simulink model "idF14Model"  (R2016a)
settings: Solver=ode45  SolverMode=SingleTasking  StartTime=0.0  StopTime=30  RelTol=1e-4  AbsTol=1e-6
PreLoadFcn:
  | g = 32.2;
  | Uo = 689.4000;
  | Vto = 690.4000;
  | % Stability derivatives
  | Mw = -0.00592;
  | Mq = -0.6571;
  | Md = -6.8847;
  | Zd = -63.9979;
  | Zw = -0.6385;
  | % Gains
  | cmdgain = 3.490954472728077e-02;
  | Ka = 0.6770;
  | Kq = 0.8156;
  | Kf = -1.7460;
  | Ki = -3.8640;
  | % Other constants
  | a = 2.5348;
  | Gamma = 0.0100;
  | b = 64.1300;
  | Beta = 426.4352;
  | Sa = 0.005236;
  | Swg = 3;
  | Ta = 0.0500;
  | Tal = 0.3959;
  | Ts = 0.0444;
  | W1 = 2.9710;
  | W2 = 4.1440;
  | Wa = 10;
libraries: simulink x1
settings Model: ExtModeTrigMode=oneshot  ExtModeArmWhenConnect=off  ExtModeAutoUpdateStatusClock=off  Creator=The MathWorks, Inc.  LastModifiedBy=The MathWorks, Inc.
settings DataIOCC: ExternalInput=[]  InitialState=[]  SaveFormat=Array  SaveOutput=off  SaveTime=off
settings OptimizationCC: BlockReduction=off  BooleanDataType=off  ExpressionDepthLimit=2147483647  InitFltsAndDblsToZero=on
settings DebuggingCC: SaveWithParameterizedLinksMsg=none  UnderspecifiedInitializationDetection=Classic  MergeDetectMultiDrivingBlocksExec=none  SignalResolutionControl=TryResolveAllWithWarning  MultiTaskDSMMsg=warning  MultiTaskCondExecSysMsg=none  IntegerOverflowMsg=none  FcnCallInpInsideContextMsg=UseLocalSettings  StateNameClashWarn=warning  IntegerSaturationMsg=none
settings HardwareCC: ProdBitPerPointer=32  ProdLargestAtomicFloat=None  ProdIntDivRoundTo=Undefined  ProdEndianess=Unspecified  ProdWordSize=32  ProdHWDeviceType=32-bit Generic
settings ModelReferenceCC: PropagateSignalLabelsOutOfModel=off
settings GRTTargetCC: TargetFcnLib=ansi_tfl_tmw.mat  CombineOutputUpdateFcns=off  GRTInterface=on
settings ConfigComp: CovModelRefEnable=Off

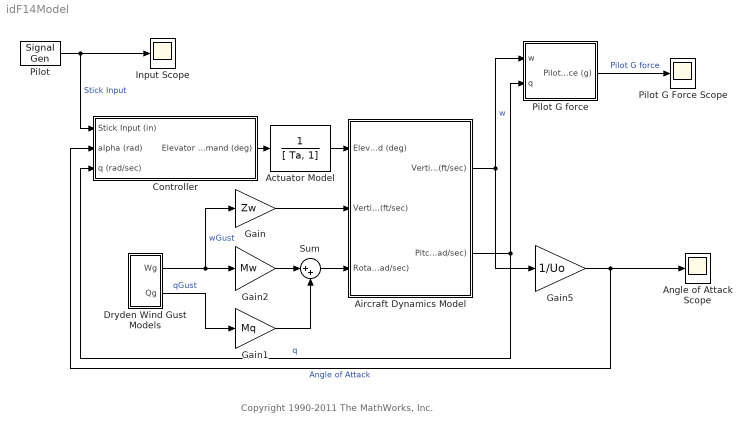
== system idF14Model ==
  note: Copyright 1990-2011 The MathWorks, Inc.
  Actuator Model : TransferFcn  Denominator=[ Ta, 1]
  Aircraft Dynamics Model : Subsystem
  Angle of Attack Scope : Scope
  Controller : Subsystem
  Dryden Wind Gust Models : Subsystem
  Gain : Gain  Gain=Zw  SaturateOnIntegerOverflow=on  OutDataTypeStr=Inherit: Same as input  ParamDataTypeStr=Inherit: Same as input
  Gain1 : Gain  Gain=Mq  SaturateOnIntegerOverflow=on  OutDataTypeStr=Inherit: Same as input  ParamDataTypeStr=Inherit: Same as input
  Gain2 : Gain  Gain=Mw  SaturateOnIntegerOverflow=on  OutDataTypeStr=Inherit: Same as input  ParamDataTypeStr=Inherit: Same as input
  Gain5 : Gain  Gain=1/Uo  SaturateOnIntegerOverflow=on  OutDataTypeStr=Inherit: Same as input  ParamDataTypeStr=Inherit: Same as input
  Input Scope : Scope
  Pilot : SignalGenerator  WaveForm=square  Frequency=0.500000  Units=rad/sec
  Pilot G Force Scope : Scope
  Pilot G force : Subsystem
  Sum : Sum  Inputs=|++  SaturateOnIntegerOverflow=on  InputSameDT=on  OutDataTypeStr=Inherit: Same as first input
  wires:
  Gain5/1 -> Angle of Attack Scope/1, Controller/2(alpha (rad))  "Angle of Attack"
  Aircraft Dynamics Model/1(Vertical Velocity w (ft/sec)) -> Gain5/1, Pilot G force/1(w)  "w"
  Pilot G force/1(Pilot g force (g)) -> Pilot G Force Scope/1  "Pilot G force"
  Gain2/1 -> Sum/1
  Gain/1 -> Aircraft Dynamics Model/2(Vertical Gust wGust (ft/sec))
  Dryden Wind Gust Models/2(Qg) -> Gain1/1  "qGust"
  Dryden Wind Gust Models/1(Wg) -> Gain2/1, Gain/1  "wGust"
  Sum/1 -> Aircraft Dynamics Model/3(Rotary Gust qGust (rad/sec))
  Gain1/1 -> Sum/2
  Aircraft Dynamics Model/2(Pitch Rate q (rad/sec)) -> Pilot G force/2(q), Controller/3(q (rad/sec))  "q"
  Actuator Model/1 -> Aircraft Dynamics Model/1(Elevator Deflection d (deg))
  Controller/1(Elevator Command (deg)) -> Actuator Model/1
  Pilot/1 -> Input Scope/1, Controller/1(Stick Input (in))  "Stick Input"

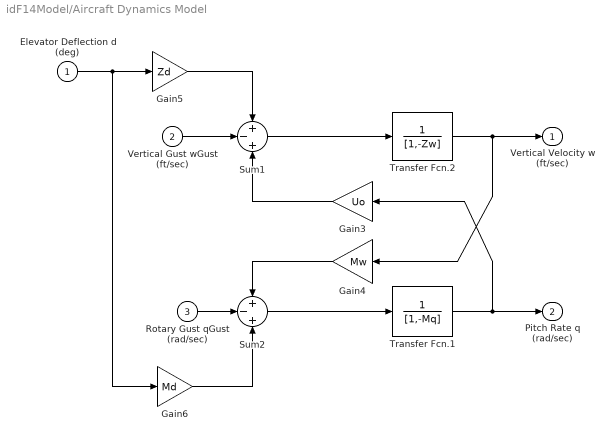
== system idF14Model/Aircraft Dynamics Model ==
  Elevator Deflection d (deg) : Inport
  Vertical Gust wGust (ft/sec) : Inport  Port=2
  Rotary Gust qGust (rad/sec) : Inport  Port=3
  Gain3 : Gain  Gain=Uo  SaturateOnIntegerOverflow=on  OutDataTypeStr=Inherit: Same as input  ParamDataTypeStr=Inherit: Same as input
  Gain4 : Gain  Gain=Mw  SaturateOnIntegerOverflow=on  OutDataTypeStr=Inherit: Same as input  ParamDataTypeStr=Inherit: Same as input
  Gain5 : Gain  Gain=Zd  SaturateOnIntegerOverflow=on  OutDataTypeStr=Inherit: Same as input  ParamDataTypeStr=Inherit: Same as input
  Gain6 : Gain  Gain=Md  SaturateOnIntegerOverflow=on  OutDataTypeStr=Inherit: Same as input  ParamDataTypeStr=Inherit: Same as input
  Sum1 : Sum  Inputs=+-+  SaturateOnIntegerOverflow=on  InputSameDT=on  OutDataTypeStr=Inherit: Same as first input
  Sum2 : Sum  Inputs=+-+  SaturateOnIntegerOverflow=on  InputSameDT=on  OutDataTypeStr=Inherit: Same as first input
  Transfer Fcn.1 : TransferFcn  Denominator=[1,-Mq]
  Transfer Fcn.2 : TransferFcn  Denominator=[1,-Zw]
  Vertical Velocity w (ft/sec) : Outport  InitialOutput=0
  Pitch Rate q (rad/sec) : Outport  Port=2  InitialOutput=0
  wires:
  Transfer Fcn.2/1 -> Vertical Velocity w (ft/sec)/1, Gain4/1
  Transfer Fcn.1/1 -> Pitch Rate q (rad/sec)/1, Gain3/1
  Gain6/1 -> Sum2/3
  Gain5/1 -> Sum1/1
  Gain3/1 -> Sum1/3
  Rotary Gust qGust (rad/sec)/1 -> Sum2/2
  Sum2/1 -> Transfer Fcn.1/1
  Sum1/1 -> Transfer Fcn.2/1
  Gain4/1 -> Sum2/1
  Vertical Gust wGust (ft/sec)/1 -> Sum1/2
  Elevator Deflection d (deg)/1 -> Gain5/1, Gain6/1

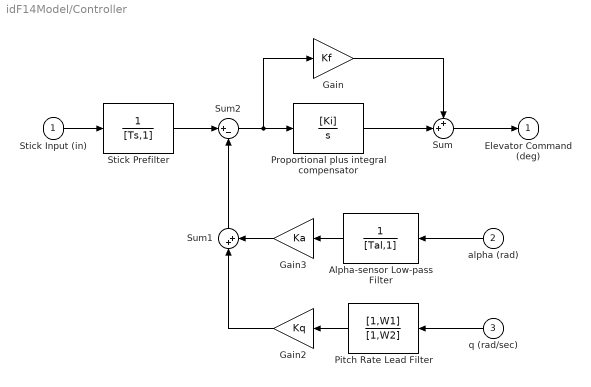
== system idF14Model/Controller ==
  Stick Input (in) : Inport
  alpha (rad) : Inport  Port=2
  q (rad/sec) : Inport  Port=3
  Alpha-sensor Low-pass Filter : TransferFcn  Denominator=[Tal,1]
  Gain : Gain  Gain=Kf  SaturateOnIntegerOverflow=on  OutDataTypeStr=Inherit: Same as input  ParamDataTypeStr=Inherit: Same as input
  Gain2 : Gain  Gain=Kq  SaturateOnIntegerOverflow=on  OutDataTypeStr=Inherit: Same as input  ParamDataTypeStr=Inherit: Same as input
  Gain3 : Gain  Gain=Ka  SaturateOnIntegerOverflow=on  OutDataTypeStr=Inherit: Same as input  ParamDataTypeStr=Inherit: Same as input
  Pitch Rate Lead Filter : TransferFcn  Numerator=[1,W1]  Denominator=[1,W2]
  Proportional plus integral compensator : TransferFcn  Numerator=[Ki]  Denominator=[1,0]
  Stick Prefilter : TransferFcn  Denominator=[Ts,1]
  Sum : Sum  Inputs=++|  SaturateOnIntegerOverflow=on  InputSameDT=on  OutDataTypeStr=Inherit: Same as first input
  Sum1 : Sum  Inputs=|++  SaturateOnIntegerOverflow=on  InputSameDT=on  OutDataTypeStr=Inherit: Same as first input
  Sum2 : Sum  Inputs=|+-  SaturateOnIntegerOverflow=on  InputSameDT=on  OutDataTypeStr=Inherit: Same as first input
  Elevator Command (deg) : Outport  InitialOutput=0
  wires:
  Sum2/1 -> Proportional plus integral compensator/1, Gain/1
  Gain/1 -> Sum/1
  Proportional plus integral compensator/1 -> Sum/2
  Stick Prefilter/1 -> Sum2/1
  Sum/1 -> Elevator Command (deg)/1
  Gain2/1 -> Sum1/1
  Gain3/1 -> Sum1/2
  Sum1/1 -> Sum2/2
  Pitch Rate Lead Filter/1 -> Gain2/1
  q (rad/sec)/1 -> Pitch Rate Lead Filter/1
  Alpha-sensor Low-pass Filter/1 -> Gain3/1
  alpha (rad)/1 -> Alpha-sensor Low-pass Filter/1
  Stick Input (in)/1 -> Stick Prefilter/1

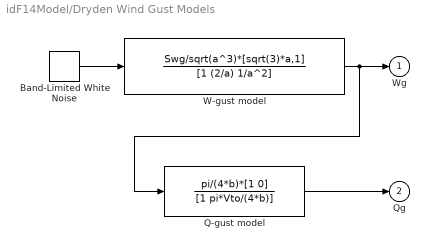
== system idF14Model/Dryden Wind Gust Models ==
  Band-Limited White Noise : simulink/Sources/Band-Limited White Noise  Cov=2  Ts=0.0444  seed=[23341]
  Q-gust model : TransferFcn  Numerator=pi/(4*b)*[1 0]  Denominator=[1 pi*Vto/(4*b)]
  W-gust model : TransferFcn  Numerator=Swg/sqrt(a^3)*[sqrt(3)*a,1]  Denominator=[1 (2/a) 1/a^2]
  Wg : Outport  InitialOutput=0
  Qg : Outport  Port=2  InitialOutput=0
  wires:
  Band-Limited White Noise/1 -> W-gust model/1
  Q-gust model/1 -> Qg/1
  W-gust model/1 -> Wg/1, Q-gust model/1

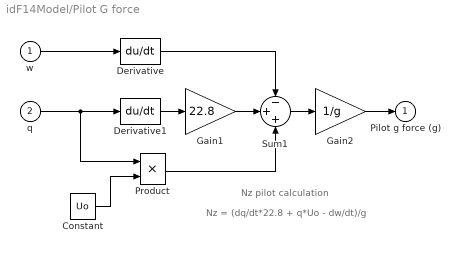
== system idF14Model/Pilot G force ==
  note: Nz pilot calculation
  note: Nz = (dq/dt*22.8 + q*Uo - dw/dt)/g
  w : Inport
  q : Inport  Port=2
  Constant : Constant  Value=Uo
  Derivative : Derivative  CoefficientInTFapproximation=1e-5
  Derivative1 : Derivative  CoefficientInTFapproximation=1e-5
  Gain1 : Gain  Gain=22.8  SaturateOnIntegerOverflow=on  OutDataTypeStr=Inherit: Same as input  ParamDataTypeStr=Inherit: Same as input
  Gain2 : Gain  Gain=1/g  SaturateOnIntegerOverflow=on  OutDataTypeStr=Inherit: Same as input  ParamDataTypeStr=Inherit: Same as input
  Product : Product  SaturateOnIntegerOverflow=on  RndMeth=Zero  InputSameDT=on  OutDataTypeStr=Inherit: Same as first input
  Sum1 : Sum  Inputs=-++  SaturateOnIntegerOverflow=on  InputSameDT=on  OutDataTypeStr=Inherit: Same as first input
  Pilot g force (g) : Outport  InitialOutput=0
  wires:
  q/1 -> Product/1, Derivative1/1
  Constant/1 -> Product/2
  Gain2/1 -> Pilot g force (g)/1
  Sum1/1 -> Gain2/1
  Derivative1/1 -> Gain1/1
  Gain1/1 -> Sum1/2
  Product/1 -> Sum1/3
  Derivative/1 -> Sum1/1
  w/1 -> Derivative/1
